simulink model "mmcs_s2f"  (R2021b)
settings: Solver=FixedStepDiscrete  StartTime=0.0  StopTime=5  FixedStep=T_HF_TASK  RelTol=1e-3  EnableMultiTasking=on
PostLoadFcn:
  | run('init.m')
values from neighbouring files (symbols this model uses):
  ALIGN_DURATION = 700.0    [mmcs_s2f_dd.sldd]
  ALIGN_FINAL_CURRENT = 3277.0    [mmcs_s2f_dd.sldd]
  ALIGN_FINAL_SPEED = 0.0    [mmcs_s2f_dd.sldd]
  ALIGN_INIT_CURRENT = 1638.0    [mmcs_s2f_dd.sldd]
  ALIGN_THETA = 2731.0    [mmcs_s2f_dd.sldd]
  AMPTOS16 = 3277.0    [mmcs_s2f_dd.sldd]
  DIVSQRT_3 = 18918.0    [mmcs_s2f_dd.sldd]
  ENC_PT_CTRL = 4.0    [mmcs_s2f_dd.sldd]
  ENC_PULSE_NUM = 4000    [mmcs_s2f_dd.sldd]
  ENC_ST_CTRL = 2.0    [mmcs_s2f_dd.sldd]
  IF_ACC_DURATION = 1500.0    [mmcs_s2f_dd.sldd]
  IF_FINAL_CURRENT = 3277.0    [mmcs_s2f_dd.sldd]
  IF_FINAL_CURRENT_LOL = -3277.0    [mmcs_s2f_dd.sldd]
  IF_FINAL_CURRENT_UPL = 3277.0    [mmcs_s2f_dd.sldd]
  IF_FINAL_SPEED = 600.0    [mmcs_s2f_dd.sldd]
  IF_FINAL_SPEED_LOL = -600.0    [mmcs_s2f_dd.sldd]
  IF_FINAL_SPEED_UPL = 600.0    [mmcs_s2f_dd.sldd]
  IF_INIT_CURRENT = 1638.0    [mmcs_s2f_dd.sldd]
  INT16_MAX = 32767.0    [mmcs_s2f_dd.sldd]
  INT16_MIN = -32768.0    [mmcs_s2f_dd.sldd]
  MOTOR_F = 7.0E-6    [mmcs_s2f_dd.sldd]
  MOTOR_J = 2.8E-6    [mmcs_s2f_dd.sldd]
  MOTOR_PN = 4    [mmcs_s2f_dd.sldd]
  MOTOR_PNF = 4.0    [mmcs_s2f_dd.sldd]
  MOTOR_TL = 0.001    [mmcs_s2f_dd.sldd]
  PI_KI_PLL : value not decoded    [mmcs_s2f_dd.sldd]
  PI_KI_POS : value not decoded    [mmcs_s2f_dd.sldd]
  PI_KI_SPD : value not decoded    [mmcs_s2f_dd.sldd]
  PI_KI_TQ : value not decoded    [mmcs_s2f_dd.sldd]
  PI_KP_PLL : value not decoded    [mmcs_s2f_dd.sldd]
  PI_KP_POS : value not decoded    [mmcs_s2f_dd.sldd]
  PI_KP_SPD : value not decoded    [mmcs_s2f_dd.sldd]
  PI_KP_TQ : value not decoded    [mmcs_s2f_dd.sldd]
  PWM_FREQUENCY = 10000.0    [mmcs_s2f_dd.sldd]
  PWM_PERIOD_CYCLES = 7200.0    [mmcs_s2f_dd.sldd]
  RAD2RPM_F_DEN = 1000.0    [mmcs_s2f_dd.sldd]
  RAD2RPM_F_NUM = 9549.0    [mmcs_s2f_dd.sldd]
  RADTOS16_F = 10430.378350470453    [mmcs_s2f_dd.sldd]
  RADTOS16_I = 10430.0    [mmcs_s2f_dd.sldd]
  REF_CURRENT_LOL = -11470.0    [mmcs_s2f_dd.sldd]
  REF_CURRENT_UPL = 11470.0    [mmcs_s2f_dd.sldd]
  STM_ALIGN = 4.0    [mmcs_s2f_dd.sldd]
  STM_IFRUN = 5.0    [mmcs_s2f_dd.sldd]
  STM_INIT = 1.0    [mmcs_s2f_dd.sldd]
  STM_PTRUN = 7.0    [mmcs_s2f_dd.sldd]
  STM_START = 12.0    [mmcs_s2f_dd.sldd]
  STM_STRUN = 6.0    [mmcs_s2f_dd.sldd]
  STM_SWITCH = 11.0    [mmcs_s2f_dd.sldd]
  STO_C1 = 588    [mmcs_s2f_dd.sldd]
  STO_C2 = -5703    [mmcs_s2f_dd.sldd]
  STO_C3 = 1554    [mmcs_s2f_dd.sldd]
  STO_C4 = 7484    [mmcs_s2f_dd.sldd]
  STO_C5 = 1831    [mmcs_s2f_dd.sldd]
  STO_EST_MAX = 134213632.0    [mmcs_s2f_dd.sldd]
  STO_EST_MIN = -134213632.0    [mmcs_s2f_dd.sldd]
  STO_F1 = 4096.0    [mmcs_s2f_dd.sldd]
  STO_F2 = 4096.0    [mmcs_s2f_dd.sldd]
  STO_ST_CTRL = 3.0    [mmcs_s2f_dd.sldd]
  STOMS = 1000.0    [mmcs_s2f_dd.sldd]
  T_HF_TASK = 0.0001    [mmcs_s2f_dd.sldd]
  T_MF_TASK = 0.002    [mmcs_s2f_dd.sldd]
  TORQ_CTRL = 0.0    [mmcs_s2f_dd.sldd]
  U32MAXdivPulseNumber = 1073741    [mmcs_s2f_dd.sldd]
  VBUS = 24.0    [mmcs_s2f_dd.sldd]
undefined symbols (not defined in the file or in its folder): DiscIntNeverNeededParam
libraries: simulink x22, slpidlib x5, mcbplantlib x1, autolibpmsmexterior x1
(part 2 of 5)

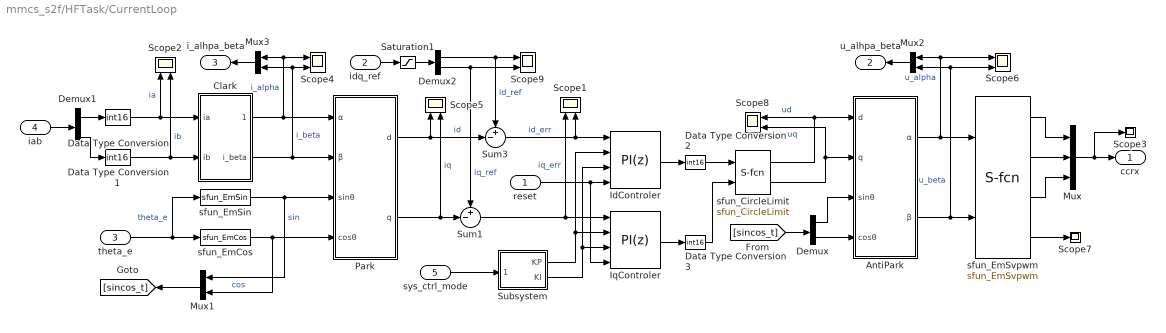
== system mmcs_s2f/HFTask/CurrentLoop ==
  reset : Inport  OutDataTypeStr=uint8
  idq_ref : Inport  Port=2
  theta_e : Inport  Port=3  OutDataTypeStr=int16
  iab : Inport  Port=4
  sys_ctrl_mode : Inport  Port=5  OutDataTypeStr=uint8
  AntiPark : Subsystem
      settings: RTWFcnNameOpts=Use subsystem name  RTWFileNameOpts=Use subsystem name
  Clark : Subsystem
      settings: RTWFcnNameOpts=Use subsystem name  RTWFileNameOpts=Use subsystem name
  Data Type Conversion{,1..3} (4 alike) : DataTypeConversion  OutDataTypeStr=int16  RndMeth=Zero
  Demux : Demux  Outputs=2
      settings: DisplayOption=none
  Demux1 : Demux  Outputs=2
      settings: DisplayOption=none
  Demux2 : Demux  Outputs=2
      settings: DisplayOption=none
  IdControler : slpidlib/PID Controller  Controller=PI  Form=Parallel  TimeDomain=Discrete-time  UseExternalTs=off  SampleTime=-1  IntegratorMethod=Forward Euler  FilterMethod=Forward Euler  ControllerParametersSource=external  P=PI_KP_TQ  I=PI_KI_TQ  D=0  UseFilter=on  N=100  TunerSelectOption=Transfer Function Based (PID Tuner App)  InitialConditionSource=internal  InitialConditionForIntegrator=0  InitialConditionForFilter=0  DifferentiatorICPrevScaledInput=0  ExternalReset=rising  TrackingMode=off  Kt=1  LimitOutput=on  SatLimitsSource=internal  UpperSaturationLimit=INT16_MAX  LowerSaturationLimit=INT16_MIN  LinearizeAsGain=off  AntiWindupMode=clamping  Kb=1  RndMeth=Zero  SaturateOnIntegerOverflow=on  PGainOutDataTypeStr=fixdt(1,32,7)  PProdOutDataTypeStr=fixdt(1,32,7)  POutMin=[]  POutMax=[]  IGainOutDataTypeStr=fixdt(1,32,7)  IProdOutDataTypeStr=fixdt(1,32,7)  IOutMin=[]  IOutMax=[]  DOutMin=[]  DOutMax=[]  NOutMin=[]  NOutMax=[]  SumOutDataTypeStr=int32  SumOutMin=[]  SumOutMax=[]  SaturationOutDataTypeStr=int32  SaturationOutMin=[]  SaturationOutMax=[]  PParamDataTypeStr=fixdt(1,32,16)  PParamMin=[]  PParamMax=[]  IParamDataTypeStr=fixdt(1,32,16)  IParamMin=[]  IParamMax=[]  DParamMin=[]  DParamMax=[]  NParamMin=[]  NParamMax=[]  KbParamMin=[]  KbParamMax=[]  KtParamMin=[]  KtParamMax=[]  KbOutMin=[]  KbOutMax=[]  KtOutMin=[]  KtOutMax=[]  IntegratorOutDataTypeStr=fixdt(1,32,7)  IntegratorOutMin=[]  IntegratorOutMax=[]  FilterOutMin=[]  FilterOutMax=[]  SumI1OutMin=[]  SumI1OutMax=[]  SumI2OutMin=[]  SumI2OutMax=[]  SumI3OutMin=[]  SumI3OutMax=[]  SumI4OutMin=[]  SumI4OutMax=[]  SumDOutMin=[]  SumDOutMax=[]  SumAccumDataTypeStr=fixdt(1,32,7)  DifferentiatorOutMin=[]  DifferentiatorOutMax=[]  FilterDiffOutCoefMin=[]  FilterDiffOutCoefMax=[]  ReciprocalOutMin=[]  ReciprocalOutMax=[]  SumDenOutMin=[]  SumDenOutMax=[]  SumNumOutMin=[]  SumNumOutMax=[]  DivideOutMin=[]  DivideOutMax=[]  UdiffTsProdOutMin=[]  UdiffTsProdOutMax=[]  NTsProdOutMin=[]  NTsProdOutMax=[]  UintegralTsProdOutMin=[]  UintegralTsProdOutMax=[]  UngainTsProdOutMin=[]  UngainTsProdOutMax=[]  IntegratorContinuousStateAttributes=''  IntegratorStateMustResolveToSignalObject=off  IntegratorRTWStateStorageClass=Auto  FilterContinuousStateAttributes=''  FilterStateMustResolveToSignalObject=off  FilterRTWStateStorageClass=Auto  ParallelPVariant=ExternalParameters  IdealPVariant=Disabled  IVariant=ExternalParameters  DVariant=Disabled  IntegratorVariant=Discrete  SatVariant=Enabled  AWVariant=DiscClampingParallel  PCopyVariant=Disabled  TRVariant=Disabled  FdbkBlocksVariant=Forward  IdealPFdbkVariant=Disabled  SatFdbkVariant=Disabled  DerivativeFilterVariant=Disabled  NVariant=Disabled  NCopyVariant=Disabled_SignalSpec  FilterICVariant=Disabled  IntegratorICVariant=InternalICs  ExternalResetVariant=ExternalReset  TRSumVariant=Passthrough  SumFdbkVariant=Disabled  SumVariant=Sum_PI  TsampFilterVariant=InternalTs  TsampNgainVariant=Passthrough  TsampIntegralVariant=Passthrough  ExternalSaturationOutDataTypeStr=Inherit: Same as second input
  IqControler : slpidlib/PID Controller  Controller=PI  Form=Parallel  TimeDomain=Discrete-time  UseExternalTs=off  SampleTime=-1  IntegratorMethod=Forward Euler  FilterMethod=Forward Euler  ControllerParametersSource=external  P=PI_KP_TQ  I=PI_KI_TQ  D=0  UseFilter=on  N=100  TunerSelectOption=Transfer Function Based (PID Tuner App)  InitialConditionSource=internal  InitialConditionForIntegrator=0  InitialConditionForFilter=0  DifferentiatorICPrevScaledInput=0  ExternalReset=rising  TrackingMode=off  Kt=1  LimitOutput=on  SatLimitsSource=internal  UpperSaturationLimit=INT16_MAX  LowerSaturationLimit=INT16_MIN  LinearizeAsGain=off  AntiWindupMode=clamping  Kb=1  RndMeth=Zero  SaturateOnIntegerOverflow=on  PGainOutDataTypeStr=fixdt(1,32,7)  PProdOutDataTypeStr=fixdt(1,32,7)  POutMin=[]  POutMax=[]  IGainOutDataTypeStr=fixdt(1,32,7)  IProdOutDataTypeStr=fixdt(1,32,7)  IOutMin=[]  IOutMax=[]  DOutMin=[]  DOutMax=[]  NOutMin=[]  NOutMax=[]  SumOutDataTypeStr=int32  SumOutMin=[]  SumOutMax=[]  SaturationOutDataTypeStr=int32  SaturationOutMin=[]  SaturationOutMax=[]  PParamDataTypeStr=fixdt(1,32,16)  PParamMin=[]  PParamMax=[]  IParamDataTypeStr=fixdt(1,32,16)  IParamMin=[]  IParamMax=[]  DParamMin=[]  DParamMax=[]  NParamMin=[]  NParamMax=[]  KbParamMin=[]  KbParamMax=[]  KtParamMin=[]  KtParamMax=[]  KbOutMin=[]  KbOutMax=[]  KtOutMin=[]  KtOutMax=[]  IntegratorOutDataTypeStr=fixdt(1,32,7)  IntegratorOutMin=[]  IntegratorOutMax=[]  FilterOutMin=[]  FilterOutMax=[]  SumI1OutMin=[]  SumI1OutMax=[]  SumI2OutMin=[]  SumI2OutMax=[]  SumI3OutMin=[]  SumI3OutMax=[]  SumI4OutMin=[]  SumI4OutMax=[]  SumDOutMin=[]  SumDOutMax=[]  SumAccumDataTypeStr=fixdt(1,32,7)  DifferentiatorOutMin=[]  DifferentiatorOutMax=[]  FilterDiffOutCoefMin=[]  FilterDiffOutCoefMax=[]  ReciprocalOutMin=[]  ReciprocalOutMax=[]  SumDenOutMin=[]  SumDenOutMax=[]  SumNumOutMin=[]  SumNumOutMax=[]  DivideOutMin=[]  DivideOutMax=[]  UdiffTsProdOutMin=[]  UdiffTsProdOutMax=[]  NTsProdOutMin=[]  NTsProdOutMax=[]  UintegralTsProdOutMin=[]  UintegralTsProdOutMax=[]  UngainTsProdOutMin=[]  UngainTsProdOutMax=[]  IntegratorContinuousStateAttributes=''  IntegratorStateMustResolveToSignalObject=off  IntegratorRTWStateStorageClass=Auto  FilterContinuousStateAttributes=''  FilterStateMustResolveToSignalObject=off  FilterRTWStateStorageClass=Auto  ParallelPVariant=ExternalParameters  IdealPVariant=Disabled  IVariant=ExternalParameters  DVariant=Disabled  IntegratorVariant=Discrete  SatVariant=Enabled  AWVariant=DiscClampingParallel  PCopyVariant=Disabled  TRVariant=Disabled  FdbkBlocksVariant=Forward  IdealPFdbkVariant=Disabled  SatFdbkVariant=Disabled  DerivativeFilterVariant=Disabled  NVariant=Disabled  NCopyVariant=Disabled_SignalSpec  FilterICVariant=Disabled  IntegratorICVariant=InternalICs  ExternalResetVariant=ExternalReset  TRSumVariant=Passthrough  SumFdbkVariant=Disabled  SumVariant=Sum_PI  TsampFilterVariant=InternalTs  TsampNgainVariant=Passthrough  TsampIntegralVariant=Passthrough  ExternalSaturationOutDataTypeStr=Inherit: Same as second input
  Mux : Mux  Inputs=3
  Mux1 : Mux  Inputs=2
  Mux2 : Mux  Inputs=2
  Mux3 : Mux  Inputs=2
  Park : Subsystem
      settings: RTWFcnNameOpts=Use subsystem name  RTWFileNameOpts=Use subsystem name
  Saturation1 : Saturate  UpperLimit=REF_CURRENT_UPL  LowerLimit=REF_CURRENT_LOL  OutDataTypeStr=int16  RndMeth=Zero
  Scope{1..2,4..6,8..9} (7 alike) : Scope  NumInputPorts=2
  Scope3 : Scope
  Scope7 : Scope
  Subsystem : Subsystem
  Sum1 : Sum  Inputs=+-|  RndMeth=Zero
  Sum3 : Sum  Inputs=+-|  RndMeth=Zero
  sfun_CircleLimit : S-Function  FunctionName=sfun_CircleLimit  SFunctionDeploymentMode=off  EnableBusSupport=off  mask(Legacy Function){SFunctionSpec=void CircleLimit(int16 u1, int16 u2, int16 y1[1], int16 y2[1]), ShowSpec=on}
      mask prompts: ShowSpec "显示函数设定"
      mask help:
      | 此模块允许您调用由以下代码继承工具定义指定的已有函数:
      | def.SFunctionName = 'sfun_CircleLimit';
      | def.OutputFcnSpec = 'void CircleLimit(int16 u1, int16 u2, int16 y1[1], int16 y2[1])';
      | def.HeaderFiles = {'circle_limit.h'};
      mask Help: <p>此模块是由代码继承工具自动生成的。有关此工具的详细帮助，请调用<a href="matlab:legacy_code('help')"> legacy_code('help')</a>.</p>
      mask Callback ShowSpec:
      | if strcmp(get_param(gcbh, 'ShowSpec'), 'on')
      |   set_param(gcbh, 'MaskDisplay', sprintf('fprintf(''%s'');', get_param(gcbh, 'SFunctionSpec')));
      | else
      |   set_param(gcbh, 'MaskDisplay', sprintf('fprintf(''%s'');', get_param(gcbh, 'FunctionName')));
      | end
      mask Display: fprintf('void CircleLimit(int16 u1, int16 u2, int16 y1[1], int16 y2[1])');
  sfun_EmCos : S-Function  FunctionName=sfun_EmCos  SFunctionDeploymentMode=off  EnableBusSupport=off  mask(Legacy Function){SFunctionSpec=int16 y1 = EmCos( int16 u1 ), ShowSpec=on}
      mask prompts: ShowSpec "显示函数设定"
      mask help:
      | 此模块允许您调用由以下代码继承工具定义指定的已有函数:
      | def.SFunctionName = 'sfun_EmCos';
      | def.OutputFcnSpec = 'int16 y1 = EmCos( int16 u1 )';
      | def.HeaderFiles = {'em_sincos.h'};
      | def.SourceFiles = {'em_sincos.c'};
      | def.IncPaths = {'.\c_code'};
      mask Help: <p>此模块是由代码继承工具自动生成的。有关此工具的详细帮助，请调用<a href="matlab:legacy_code('help')"> legacy_code('help')</a>.</p>
      mask Callback ShowSpec:
      | if strcmp(get_param(gcbh, 'ShowSpec'), 'on')
      |   set_param(gcbh, 'MaskDisplay', sprintf('fprintf(''%s'');', get_param(gcbh, 'SFunctionSpec')));
      | else
      |   set_param(gcbh, 'MaskDisplay', sprintf('fprintf(''%s'');', get_param(gcbh, 'FunctionName')));
      | end
      mask Display: fprintf('int16 y1 = EmCos( int16 u1 )');
  sfun_EmSin : S-Function  FunctionName=sfun_EmSin  SFunctionDeploymentMode=off  EnableBusSupport=off  mask(Legacy Function){SFunctionSpec=int16 y1 = EmSin( int16 u1 ), ShowSpec=on}
      mask prompts: ShowSpec "显示函数设定"
      mask help:
      | 此模块允许您调用由以下代码继承工具定义指定的已有函数:
      | def.SFunctionName = 'sfun_EmSin';
      | def.OutputFcnSpec = 'int16 y1 = EmSin( int16 u1 )';
      | def.HeaderFiles = {'em_sincos.h'};
      | def.SourceFiles = {'em_sincos.c'};
      | def.IncPaths = {'.\c_code'};
      mask Help: <p>此模块是由代码继承工具自动生成的。有关此工具的详细帮助，请调用<a href="matlab:legacy_code('help')"> legacy_code('help')</a>.</p>
      mask Callback ShowSpec:
      | if strcmp(get_param(gcbh, 'ShowSpec'), 'on')
      |   set_param(gcbh, 'MaskDisplay', sprintf('fprintf(''%s'');', get_param(gcbh, 'SFunctionSpec')));
      | else
      |   set_param(gcbh, 'MaskDisplay', sprintf('fprintf(''%s'');', get_param(gcbh, 'FunctionName')));
      | end
      mask Display: fprintf('int16 y1 = EmSin( int16 u1 )');
  sfun_EmSvpwm : S-Function  FunctionName=sfun_EmSvpwm  SFunctionDeploymentMode=off  EnableBusSupport=off  mask(Legacy Function){SFunctionSpec=void EmSvpwm(int16 u1, int16 u2, uint16 y1[1], uint16 y2[1], uint16 y3[1], uint16 y4[1]), ShowSpec=on}
      mask prompts: ShowSpec "显示函数设定"
      mask help:
      | 此模块允许您调用由以下代码继承工具定义指定的已有函数:
      | def.SFunctionName = 'sfun_EmSvpwm';
      | def.OutputFcnSpec = 'void EmSvpwm(int16 u1, int16 u2, uint16 y1[1], uint16 y2[1], uint16 y3[1], uint16 y4[1])';
      | def.HeaderFiles = {'em_svpwm.h'};
      | def.SourceFiles = {'em_svpwm.c'};
      | def.IncPaths = {'..\code\MATLAB'};
      mask Help: <p>此模块是由代码继承工具自动生成的。有关此工具的详细帮助，请调用<a href="matlab:legacy_code('help')"> legacy_code('help')</a>.</p>
      mask Callback ShowSpec:
      | if strcmp(get_param(gcbh, 'ShowSpec'), 'on')
      |   set_param(gcbh, 'MaskDisplay', sprintf('fprintf(''%s'');', get_param(gcbh, 'SFunctionSpec')));
      | else
      |   set_param(gcbh, 'MaskDisplay', sprintf('fprintf(''%s'');', get_param(gcbh, 'FunctionName')));
      | end
      mask Display: fprintf('void EmSvpwm(int16 u1, int16 u2, uint16 y1[1], uint16 y2[1], uint16 y3[1], uint16 y4[1])');
  ccrx : Outport
  u_alhpa_beta : Outport  Port=2  OutDataTypeStr=int16
  i_alhpa_beta : Outport  Port=3  OutDataTypeStr=int16
  wires:
  Park/2(q) -> Sum1/2, Scope5/2  "iq"
  Sum1/1 -> IqControler/1, Scope1/1  "iq_err"
  Clark/2(i_beta) -> Scope4/2, Mux3/2, Park/2(β)  "i_beta"
  Park/1(d) -> Sum3/2, Scope5/1  "id"
  Sum3/1 -> IdControler/1, Scope1/2  "id_err"
  iab/1 -> Demux1/1
  Demux2/1 -> Scope9/1, Sum3/1  "id_ref"
  Demux2/2 -> Scope9/2, Sum1/1  "iq_ref"
  sfun_EmSin/1 -> Mux1/1, Park/3(sinθ)  "sin"
  sfun_EmCos/1 -> Park/4(cosθ), Mux1/2  "cos"
  IqControler/1 -> Data Type Conversion3/1
  IdControler/1 -> Data Type Conversion2/1
  AntiPark/2(β) -> Scope6/2, Mux2/2, sfun_EmSvpwm/2  "u_beta"
  sfun_EmSvpwm/4 -> Scope7/1
  AntiPark/1(α) -> Scope6/1, Mux2/1, sfun_EmSvpwm/1  "u_alpha"
  sfun_EmSvpwm/2 -> Mux/2
  sfun_EmSvpwm/1 -> Mux/1
  Mux/1 -> Scope3/1, ccrx/1
  sfun_EmSvpwm/3 -> Mux/3
  Mux1/1 -> [sincos_t]
  [sincos_t] -> Demux/1
  Demux/2 -> AntiPark/4(cosθ)
  Demux/1 -> AntiPark/3(sinθ)
  Clark/1(i_alpha) -> Scope4/1, Mux3/1, Park/1(α)  "i_alpha"
  Data Type Conversion/1 -> Scope2/1, Clark/1(ia)  "ia"
  Demux1/2 -> Data Type Conversion1/1
  Data Type Conversion1/1 -> Scope2/2, Clark/2(ib)  "ib"
  theta_e/1 -> sfun_EmSin/1, sfun_EmCos/1  "theta_e"
  sfun_CircleLimit/1 -> Scope8/1, AntiPark/1(d)  "ud"
  sfun_CircleLimit/2 -> AntiPark/2(q), Scope8/2  "uq"
  reset/1 -> IqControler/4, IdControler/4
  Mux2/1 -> u_alhpa_beta/1
  Mux3/1 -> i_alhpa_beta/1
  Demux1/1 -> Data Type Conversion/1
  idq_ref/1 -> Saturation1/1
  Data Type Conversion2/1 -> sfun_CircleLimit/1
  Data Type Conversion3/1 -> sfun_CircleLimit/2
  Saturation1/1 -> Demux2/1
  Subsystem/2(KI) -> IdControler/3, IqControler/3
  Subsystem/1(KP) -> IdControler/2, IqControler/2
  sys_ctrl_mode/1 -> Subsystem/1(mode)

== system mmcs_s2f/HFTask/ObserverPLL ==
  reset_all : Inport  OutDataTypeStr=uint8
  u_alpha_beta : Inport  Port=2  OutDataTypeStr=int16
  i_alpha_beta : Inport  Port=3  OutDataTypeStr=int16
  reset : Inport  Port=4  OutDataTypeStr=uint8
  spd_ref : Inport  Port=5  OutDataTypeStr=int16
  Action Port : ActionPort  ActionPortLabel=if(u1 > 0)
  Resettable Subsystem : Subsystem  TreatAsAtomicUnit=on
  theta_e_dot : Outport  OutDataTypeStr=int16
  w_dot : Outport  Port=2  OutDataTypeStr=int16
  iα_dot_next : Outport  Port=3  OutDataTypeStr=int32
  iβ_dot_next : Outport  Port=4  OutDataTypeStr=int32
  wires:
  u_alpha_beta/1 -> Resettable Subsystem/1(u_alpha_beta)
  i_alpha_beta/1 -> Resettable Subsystem/2(i_alpha_beta)
  reset/1 -> Resettable Subsystem/3(reset)
  spd_ref/1 -> Resettable Subsystem/4(spd_ref)
  Resettable Subsystem/1(theta_e_dot) -> theta_e_dot/1
  Resettable Subsystem/2(w_dot) -> w_dot/1
  Resettable Subsystem/3(iα_dot_next) -> iα_dot_next/1
  Resettable Subsystem/4(iβ_dot_next) -> iβ_dot_next/1
  reset_all/1 -> Resettable Subsystem/Reset

== system mmcs_s2f/Inverter_PMSM/Tabc2Dabc ==
  note: Dabc = Tabc / ((PWM_PERIOD_CYCLES) / 2)
  Tabc : Inport  OutDataTypeStr=uint16
  Constant2 : Constant  Value=PWM_PERIOD_CYCLES  OutDataTypeStr=single
  Divide : Product  Inputs=*/
  Gain : Gain  Gain=1/2
  Dabc : Outport  OutDataTypeStr=single
  wires:
  Tabc/1 -> Divide/1
  Divide/1 -> Dabc/1
  Constant2/1 -> Gain/1
  Gain/1 -> Divide/2

== system mmcs_s2f/MFTask/IsTransition ==
  sys_ctrl_mode : Inport  OutDataTypeStr=uint8
  stm_state : Inport  Port=2  OutDataTypeStr=uint8
  spd_dot : Inport  Port=3  OutDataTypeStr=int16
  spd_ref : Inport  Port=4  OutDataTypeStr=int16
  Abs : Abs  RndMeth=Zero
  Compare To Constant : simulink/Logic and Bit Operations/Compare To Constant  relop=>=  const=IF_FINAL_SPEED  OutDataTypeStr=boolean
  Constant : Constant  Value=STO_ST_CTRL  OutDataTypeStr=uint8
  Constant1 : Constant  Value=STM_IFRUN  OutDataTypeStr=uint8
  If : If  IfExpression=u1  ShowElse=off
  If Action Subsystem : Subsystem  TreatAsAtomicUnit=on
  Logical Operator : Logic  AllPortsSameDT=off  OutDataTypeStr=boolean
  Logical Operator1 : Logic  AllPortsSameDT=off  OutDataTypeStr=boolean
  Relational Operator : RelationalOperator  Operator===  OutDataTypeStr=boolean  RndMeth=Zero
  Relational Operator1 : RelationalOperator  Operator===  OutDataTypeStr=boolean  RndMeth=Zero
  Unit Delay1 : UnitDelay  SampleTime=-1  HasFrameUpgradeWarning=on
  transition : Outport  OutDataTypeStr=boolean
  wires:
  If/1 -> If Action Subsystem/Action
  If Action Subsystem/1(transition) -> Logical Operator1/1
  Constant/1 -> Relational Operator/2
  Logical Operator/1 -> If/1
  Constant1/1 -> Relational Operator1/2
  Relational Operator1/1 -> Logical Operator/2
  Relational Operator/1 -> Logical Operator/1
  Unit Delay1/1 -> Relational Operator1/1
  stm_state/1 -> Unit Delay1/1
  sys_ctrl_mode/1 -> Relational Operator/1
  spd_dot/1 -> If Action Subsystem/1(spd_dot)
  spd_ref/1 -> Abs/1
  Abs/1 -> Compare To Constant/1
  Compare To Constant/1 -> Logical Operator1/2
  Logical Operator1/1 -> transition/1

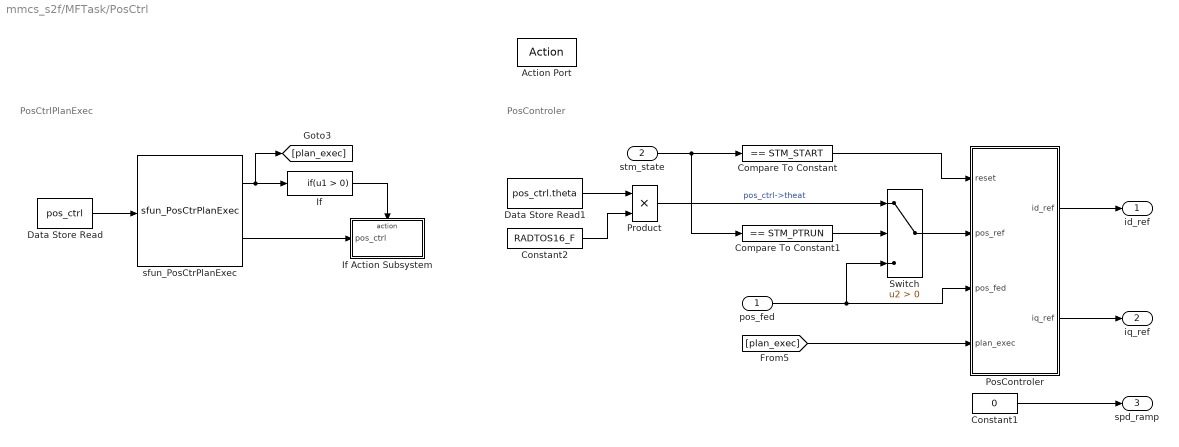
== system mmcs_s2f/MFTask/PosCtrl ==
  note: PosControler
  note: PosCtrlPlanExec
  pos_fed : Inport  OutDataTypeStr=int32
  stm_state : Inport  Port=2  OutDataTypeStr=uint8
  Action Port : ActionPort  ActionPortLabel=case [ 2 ]:
  Compare To Constant : simulink/Logic and Bit Operations/Compare To Constant  relop===  const=STM_START  OutDataTypeStr=uint8
  Compare To Constant1 : simulink/Logic and Bit Operations/Compare To Constant  relop===  const=STM_PTRUN  OutDataTypeStr=uint8
  Constant1 : Constant  Value=0  OutDataTypeStr=int16
  Constant2 : Constant  Value=RADTOS16_F  OutDataTypeStr=single
  Data Store Read : DataStoreRead  DataStoreName=pos_ctrl  DataStoreElements=pos_ctrl  IndexOptions=Index vector (dialog)  Indices=1  OutputSizes=1
  Data Store Read1 : DataStoreRead  DataStoreName=pos_ctrl  DataStoreElements=pos_ctrl.theta  IndexOptions=Index vector (dialog)  Indices=1  OutputSizes=1
  If : If  ShowElse=off
  If Action Subsystem : Subsystem  TreatAsAtomicUnit=on
  PosControler : Subsystem
  Product : Product  OutDataTypeStr=int32  RndMeth=Zero
  Switch : Switch  Criteria=u2 > Threshold  RndMeth=Zero
  sfun_PosCtrPlanExec : S-Function  FunctionName=sfun_PosCtrPlanExec  SFunctionDeploymentMode=off  EnableBusSupport=off  mask(Legacy Function){SFunctionSpec=uint8 y1 = PosCtrPlanExec(PosCtrlHandle_t u1[1], PosCtrlHandle_t y2[1]), ShowSpec=off}
      mask prompts: ShowSpec "显示函数设定"
      mask help:
      | 此模块允许您调用由以下代码继承工具定义指定的已有函数:
      | def.SFunctionName = 'sfun_PosCtrPlanExec';
      | def.OutputFcnSpec = 'uint8 y1 = PosCtrPlanExec(PosCtrlHandle_t u1[1], PosCtrlHandle_t y2[1])';
      | def.HeaderFiles = {'trajectory_ctrl.h'};
      mask Help: <p>此模块是由代码继承工具自动生成的。有关此工具的详细帮助，请调用<a href="matlab:legacy_code('help')"> legacy_code('help')</a>.</p>
      mask Callback ShowSpec:
      | if strcmp(get_param(gcbh, 'ShowSpec'), 'on')
      |   set_param(gcbh, 'MaskDisplay', sprintf('fprintf(''%s'');', get_param(gcbh, 'SFunctionSpec')));
      | else
      |   set_param(gcbh, 'MaskDisplay', sprintf('fprintf(''%s'');', get_param(gcbh, 'FunctionName')));
      | end
      mask Display: fprintf('sfun_PosCtrPlanExec');
  id_ref : Outport  OutDataTypeStr=int16
  iq_ref : Outport  Port=2  OutDataTypeStr=int16
  spd_ramp : Outport  Port=3  OutDataTypeStr=int16
  wires:
  stm_state/1 -> Compare To Constant1/1, Compare To Constant/1
  PosControler/1(id_ref) -> id_ref/1
  PosControler/2(iq_ref) -> iq_ref/1
  Constant1/1 -> spd_ramp/1
  Constant2/1 -> Product/2
  pos_fed/1 -> Switch/3, PosControler/3(pos_fed)
  Data Store Read/1 -> sfun_PosCtrPlanExec/1
  Compare To Constant1/1 -> Switch/2
  Data Store Read1/1 -> Product/1
  sfun_PosCtrPlanExec/1 -> [plan_exec], If/1
  sfun_PosCtrPlanExec/2 -> If Action Subsystem/1(pos_ctrl)
  If/1 -> If Action Subsystem/Action
  Product/1 -> Switch/1  "pos_ctrl->theat"
  Switch/1 -> PosControler/2(pos_ref)
  Compare To Constant/1 -> PosControler/1(reset)
  [plan_exec] -> PosControler/4(plan_exec)

== system mmcs_s2f/MFTask/PosCtrlInit ==
  state : Inport  OutDataTypeStr=uint8
  Compare To Constant1 : simulink/Logic and Bit Operations/Compare To Constant  relop===  const=STM_INIT  OutDataTypeStr=boolean
  If1 : If  IfExpression=u1  ShowElse=off
  PosCtrlInit : Subsystem  TreatAsAtomicUnit=on
  wires:
  If1/1 -> PosCtrlInit/Action
  Compare To Constant1/1 -> If1/1
  state/1 -> Compare To Constant1/1

== system mmcs_s2f/MFTask/PosCtrlPlan ==
  pos_fed : Inport  OutDataTypeStr=int32  LockScale=on
  pos_ref : Inport  Port=2  OutDataTypeStr=single  LockScale=on
  duration : Inport  Port=3  OutDataTypeStr=single  LockScale=on
  state : Inport  Port=4  OutDataTypeStr=uint8
  Compare To Constant3 : simulink/Logic and Bit Operations/Compare To Constant  relop===  const=STM_PTRUN  OutDataTypeStr=boolean
  Data Store Read : DataStoreRead  DataStoreName=pos_ctrl  DataStoreElements=pos_ctrl.final_angle  IndexOptions=Index vector (dialog)  Indices=1  OutputSizes=1
  If : If  IfExpression=u1  ShowElse=off
  Logical Operator1 : Logic  AllPortsSameDT=off  OutDataTypeStr=boolean
  PosCtrlPlan : Subsystem  TreatAsAtomicUnit=on
  Relational Operator : RelationalOperator  Operator=~=  OutDataTypeStr=boolean  RndMeth=Zero
  Scope : Scope  NumInputPorts=2
  wires:
  state/1 -> Compare To Constant3/1
  Relational Operator/1 -> Logical Operator1/2
  duration/1 -> PosCtrlPlan/3(duration)
  If/1 -> PosCtrlPlan/Action
  Compare To Constant3/1 -> Logical Operator1/1
  Logical Operator1/1 -> If/1
  pos_fed/1 -> PosCtrlPlan/1(pos_fed)
  pos_ref/1 -> Scope/1, PosCtrlPlan/2(pos_ref), Relational Operator/2
  Data Store Read/1 -> Scope/2, Relational Operator/1

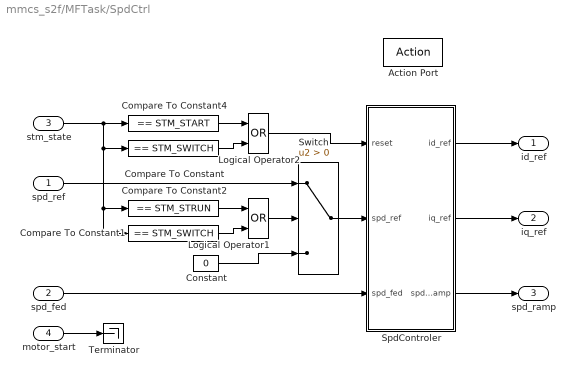
== system mmcs_s2f/MFTask/SpdCtrl ==
  spd_ref : Inport  OutDataTypeStr=int16
  spd_fed : Inport  Port=2  OutDataTypeStr=int16
  stm_state : Inport  Port=3  OutDataTypeStr=uint8
  motor_start : Inport  Port=4  OutDataTypeStr=uint8
  Action Port : ActionPort  ActionPortLabel=case [ 1 ]:
  Compare To Constant : simulink/Logic and Bit Operations/Compare To Constant  relop===  const=STM_SWITCH  OutDataTypeStr=uint8
  Compare To Constant1 : simulink/Logic and Bit Operations/Compare To Constant  relop===  const=STM_SWITCH  OutDataTypeStr=uint8
  Compare To Constant2 : simulink/Logic and Bit Operations/Compare To Constant  relop===  const=STM_STRUN  OutDataTypeStr=uint8
  Compare To Constant4 : simulink/Logic and Bit Operations/Compare To Constant  relop===  const=STM_START  OutDataTypeStr=uint8
  Constant : Constant  Value=0  OutDataTypeStr=int16
  Logical Operator1 : Logic  Operator=OR  AllPortsSameDT=off  OutDataTypeStr=boolean
  Logical Operator2 : Logic  Operator=OR  AllPortsSameDT=off  OutDataTypeStr=boolean
  SpdControler : Subsystem
  Switch : Switch  Criteria=u2 > Threshold  RndMeth=Zero
  Terminator : Terminator
  id_ref : Outport  OutDataTypeStr=int16
  iq_ref : Outport  Port=2  OutDataTypeStr=int16
  spd_ramp : Outport  Port=3  OutDataTypeStr=int16
  wires:
  Constant/1 -> Switch/3
  spd_ref/1 -> Switch/1
  SpdControler/3(spd_ramp) -> spd_ramp/1
  SpdControler/2(iq_ref) -> iq_ref/1
  Switch/1 -> SpdControler/2(spd_ref)
  Compare To Constant1/1 -> Logical Operator1/2
  spd_fed/1 -> SpdControler/3(spd_fed)
  SpdControler/1(id_ref) -> id_ref/1
  stm_state/1 -> Compare To Constant2/1, Compare To Constant1/1, Compare To Constant/1, Compare To Constant4/1
  motor_start/1 -> Terminator/1
  Compare To Constant/1 -> Logical Operator2/2
  Logical Operator1/1 -> Switch/2
  Compare To Constant2/1 -> Logical Operator1/1
  Logical Operator2/1 -> SpdControler/1(reset)
  Compare To Constant4/1 -> Logical Operator2/1
